simulink model "open_loop_second"  (R2019b)
settings: Solver=VariableStepAuto  StartTime=0.0  StopTime=400  RelTol=1e-3
values from neighbouring files (symbols this model uses):
  b = [2 2]    [test.m]
  J = 9.25 * 10^(-6)    (= 9.25e-06)    [motor_TF.m]
  Ke = 1.278    [dc_mot_p2.m]    (also in dc_mot_p3.m; motor_TF.m = 0.9549)
  L = zeros(size(V))    [Left_Pwm.m]    (also in ediff.m; mdiff.m; motor_TF.m = 0.00056)
  R = 0.1472    [dc_mot_p2.m]    (also in dc_mot_p3.m; motor_TF.m = 1.2)
  Te = (L/(3*R))    (= 0.000155555555556)    [motor_TF.m]
  Tm = (3*R*J)/(Ke*Kt)    (= 0.0013675592763)    [motor_TF.m]
undefined symbols (not defined in the file or in its folder): K
settings Model: Creator=srikesh  LastModifiedBy=srikesh

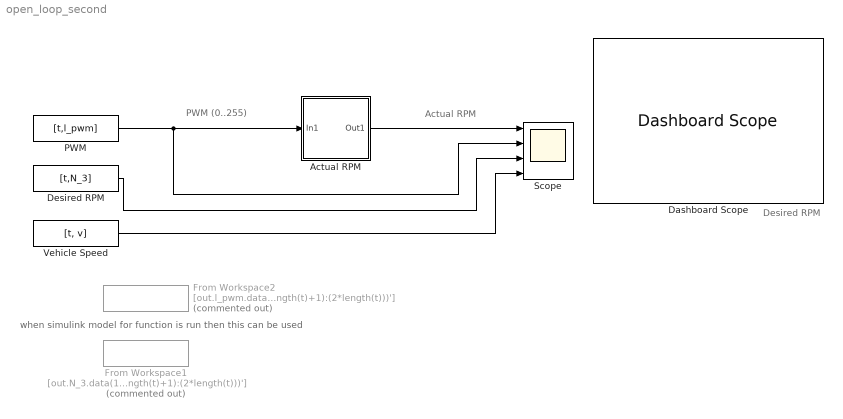
== system open_loop_second ==
  note: when simulink model for function is run then this can be used
  note: Actual RPM
  note: PWM (0..255)
  note: Desired RPM
  Actual RPM : Subsystem
  Dashboard Scope : DashboardScope
  Desired RPM : FromWorkspace  VariableName=[t,N_3]  SampleTime=0
  From Workspace1 : FromWorkspace  Commented=on  VariableName=[out.N_3.data(1:length(t))', out.N_3.data((length(t)+1):(2*length(t)))']  SampleTime=0
  From Workspace2 : FromWorkspace  Commented=on  VariableName=[out.l_pwm.data(1:length(t))', out.l_pwm.data((length(t)+1):(2*length(t)))']  SampleTime=0
  PWM : FromWorkspace  VariableName=[t,l_pwm]  SampleTime=0
  Scope : Scope  NumInputPorts=4
  "Vehicle Speed " : FromWorkspace  VariableName=[t, v]  SampleTime=0
  wires:
  "Vehicle Speed "/1 -> Scope/4
  Desired RPM/1 -> Scope/3
  PWM/1 -> Actual RPM/1(In1), Scope/2
  Actual RPM/1(Out1) -> Scope/1

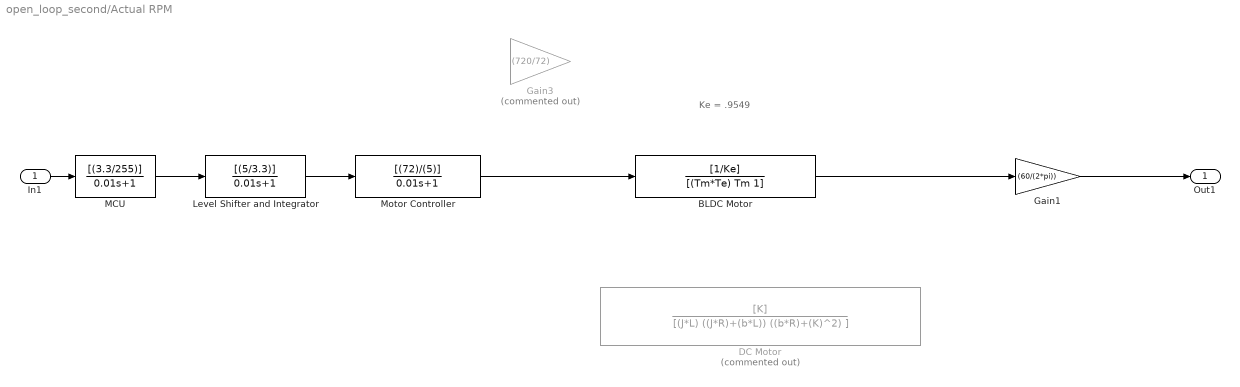
== system open_loop_second/Actual RPM ==
  note: Ke = .9549
  In1 : Inport
  BLDC Motor : TransferFcn  Numerator=[1/Ke]  Denominator=[(Tm*Te) Tm 1]
  DC Motor : TransferFcn  Commented=on  Numerator=[K]  Denominator=[(J*L) ((J*R)+(b*L)) ((b*R)+(K)^2) ]
  Gain1 : Gain  Gain=(60/(2*pi))
  Gain3 : Gain  Commented=on  Gain=(720/72)
  Level Shifter and Integrator : TransferFcn  Numerator=[(5/3.3)]  Denominator=[0.01 1]
  MCU : TransferFcn  Numerator=[(3.3/255)]  Denominator=[0.01 1]
  Motor Controller : TransferFcn  Numerator=[(72)/(5)]  Denominator=[0.01 1]
  Out1 : Outport
  wires:
  In1/1 -> MCU/1
  MCU/1 -> Level Shifter and Integrator/1
  Level Shifter and Integrator/1 -> Motor Controller/1
  Gain1/1 -> Out1/1
  Motor Controller/1 -> BLDC Motor/1
  BLDC Motor/1 -> Gain1/1
